simulink model "MODBUS_v2"  (R2019a)
settings: Solver=FixedStepAuto  StartTime=0.0  StopTime=inf  FixedStep=0.5  MaxStep=0.2  RelTol=1e-3
libraries: modbusMatLib x4, realtime_pacer_lib x1
settings Model: Creator=jvl  LastModifiedBy=pppc
settings DataIOCC: ReturnWorkspaceOutputs=off
settings DebuggingCC: PregeneratedLibrarySubsystemCodeDiagnostic=none  ArithmeticOperatorsInVariantConditions=warning
settings SFSimCC: SimUseLocalCustomCode=off
settings RTWCC: RTWUseLocalCustomCode=off

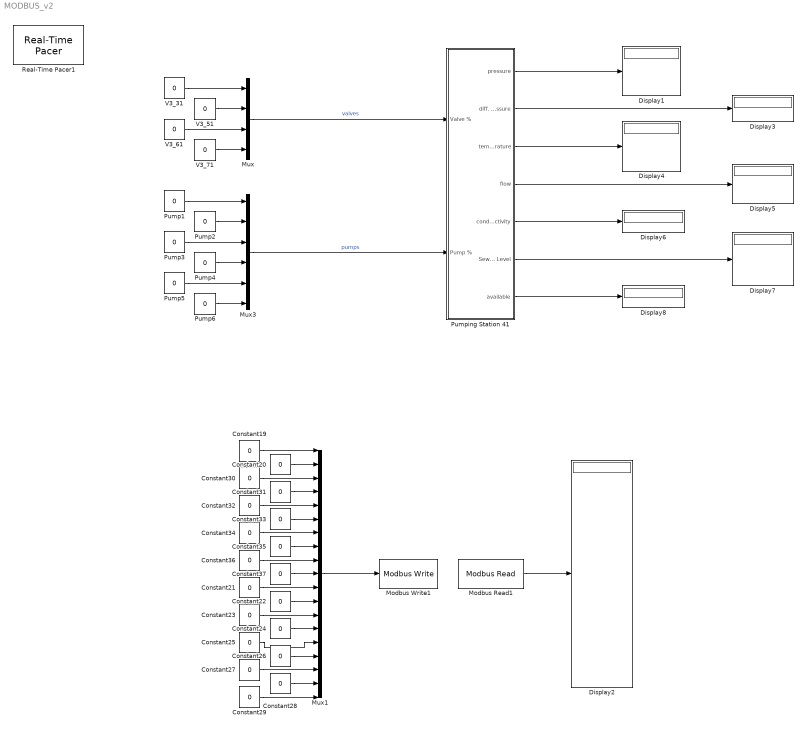
== system MODBUS_v2 ==
  Constant{19..37} (19 alike) : Constant  Value=0
  Display{1..8} (8 alike) : Display
  Modbus Read1 : modbusMatLib/Modbus Read  registry=001  ipAddress='192.168.100.30'  port=502
  Modbus Write1 : modbusMatLib/Modbus Write  registry=001  port=502  ipAddress='192.168.100.30'
  Mux : Mux
  Mux1 : Mux  Inputs=19
  Mux3 : Mux  Inputs=6
  Pump{1..6} (6 alike) : Constant  Value=0
  Pumping Station 41 : Subsystem
  Real-Time Pacer1 : realtime_pacer_lib/Real-Time Pacer  simTimePerRealTime=1
  V3_{31,51,61,71} (4 alike) : Constant  Value=0
  wires:
  V3_31/1 -> Mux/1
  V3_61/1 -> Mux/3
  V3_51/1 -> Mux/2
  V3_71/1 -> Mux/4
  Constant21/1 -> Mux1/11
  Modbus Read1/1 -> Display2/1
  Constant23/1 -> Mux1/13
  Constant31/1 -> Mux1/4
  Constant25/1 -> Mux1/15
  Constant34/1 -> Mux1/7
  Constant37/1 -> Mux1/10
  Constant33/1 -> Mux1/6
  Constant20/1 -> Mux1/2
  Constant36/1 -> Mux1/9
  Constant32/1 -> Mux1/5
  Mux1/1 -> Modbus Write1/1
  Constant26/1 -> Mux1/16
  Constant30/1 -> Mux1/3
  Constant22/1 -> Mux1/12
  Constant24/1 -> Mux1/14
  Constant35/1 -> Mux1/8
  Constant28/1 -> Mux1/18
  Constant19/1 -> Mux1/1
  Constant29/1 -> Mux1/19
  Constant27/1 -> Mux1/17
  Pump1/1 -> Mux3/1
  Pump2/1 -> Mux3/2
  Pump3/1 -> Mux3/3
  Pump4/1 -> Mux3/4
  Pump5/1 -> Mux3/5
  Pump6/1 -> Mux3/6
  Mux/1 -> Pumping Station 41/1(Valve %)  "valves"
  Mux3/1 -> Pumping Station 41/2(Pump %)  "pumps"
  Pumping Station 41/1(pressure) -> Display1/1
  Pumping Station 41/2(diff. pressure) -> Display3/1
  Pumping Station 41/3(temperature) -> Display4/1
  Pumping Station 41/4(flow) -> Display5/1
  Pumping Station 41/5(conductivity) -> Display6/1
  Pumping Station 41/6(Sewer Level) -> Display7/1
  Pumping Station 41/7(available) -> Display8/1

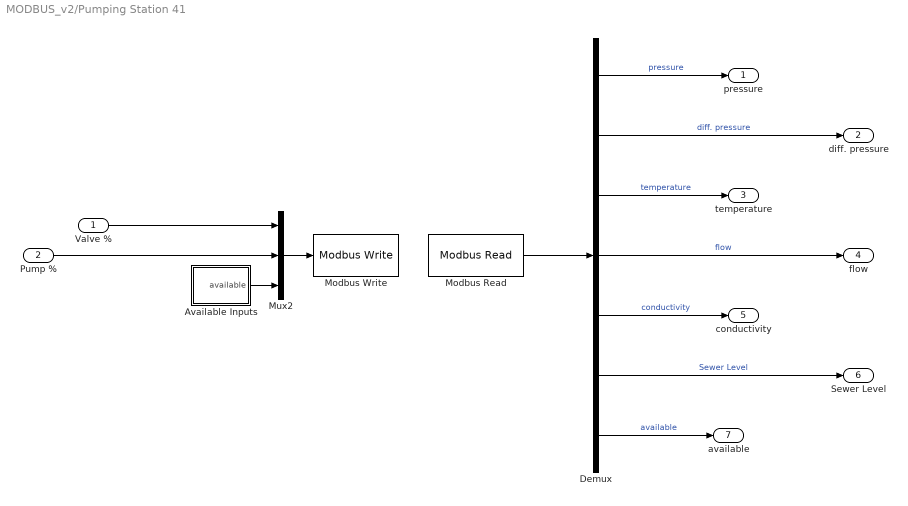
== system MODBUS_v2/Pumping Station 41 ==
  Valve % : Inport
  Pump % : Inport  Port=2
  Available Inputs : Subsystem
  Demux : Demux  Outputs=[4 2 4 3 1 4 -1]
  Modbus Read : modbusMatLib/Modbus Read  registry=001  ipAddress='192.168.100.41'  port=502
  Modbus Write : modbusMatLib/Modbus Write  registry=001  port=502  ipAddress='192.168.100.41'
  Mux2 : Mux  Inputs=3
  pressure : Outport
  diff. pressure : Outport  Port=2
  temperature : Outport  Port=3
  flow : Outport  Port=4
  conductivity : Outport  Port=5
  Sewer Level : Outport  Port=6
  available : Outport  Port=7
  wires:
  Demux/6 -> Sewer Level/1  "Sewer Level"
  Modbus Read/1 -> Demux/1
  Valve %/1 -> Mux2/1
  Available Inputs/1(available) -> Mux2/3
  Pump %/1 -> Mux2/2
  Mux2/1 -> Modbus Write/1
  Demux/5 -> conductivity/1  "conductivity"
  Demux/2 -> diff. pressure/1  "diff. pressure"
  Demux/7 -> available/1  "available"
  Demux/4 -> flow/1  "flow"
  Demux/1 -> pressure/1  "pressure"
  Demux/3 -> temperature/1  "temperature"

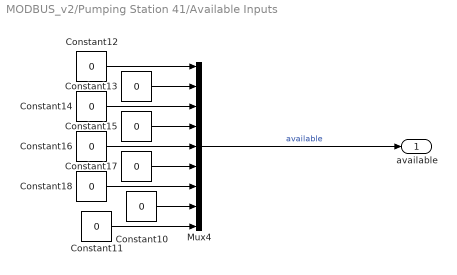
== system MODBUS_v2/Pumping Station 41/Available Inputs ==
  Constant{10..18} (9 alike) : Constant  Value=0
  Mux4 : Mux  Inputs=9
  available : Outport
  wires:
  Constant10/1 -> Mux4/8
  Constant16/1 -> Mux4/5
  Constant15/1 -> Mux4/4
  Constant18/1 -> Mux4/7
  Constant17/1 -> Mux4/6
  Constant13/1 -> Mux4/2
  Constant12/1 -> Mux4/1
  Constant11/1 -> Mux4/9
  Constant14/1 -> Mux4/3
  Mux4/1 -> available/1  "available"
